simulink model "P1Ej5"  (R2022a)
settings: Solver=VariableStepAuto  StartTime=0.0  StopTime=10.0  RelTol=1e-3
settings Model: Creator=Adrian  LastModifiedBy=Adrian

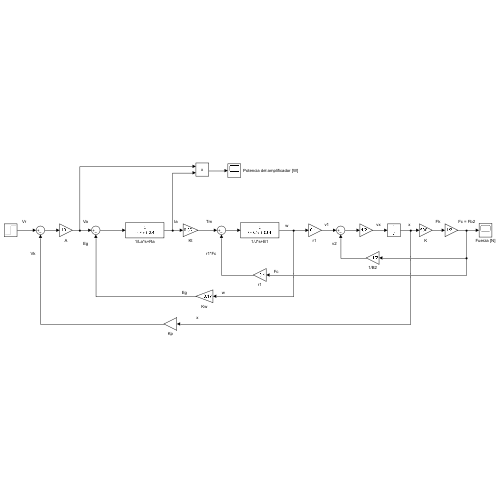
[thumbnail: Simulink's stored preview of the top-level diagram]
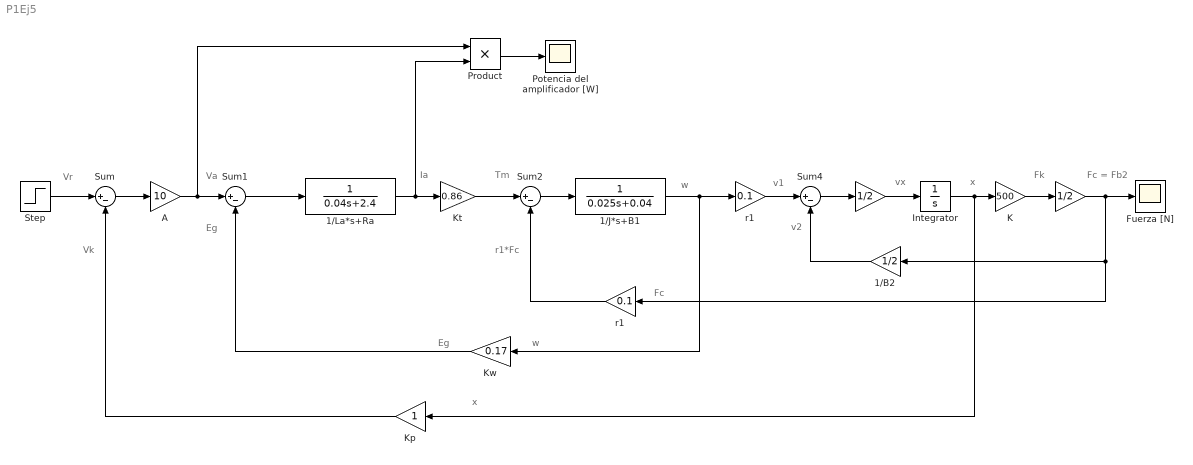
== system P1Ej5 ==
  note: vx
  note: x
  note: x
  note: v2
  note: Fk
  note: v1
  note: w
  note: Eg
  note: w
  note: Fc
  note: r1*Fc
  note: Tm
  note: Ia
  note: Eg
  note: Va
  note: Vk
  note: Fc = Fb2
  note: Vr
  " " : Gain  Gain=1/2
  "   " : Gain  Gain=1/2
  1/B2 : Gain  Gain=1/2
  1/J*s+B1 : TransferFcn  Denominator=[0.025 0.04]
  1/La*s+Ra : TransferFcn  Denominator=[0.04 2.4]
  A : Gain  Gain=10
  Fuerza [N] : Scope
  Integrator : Integrator
  K : Gain  Gain=500
  Kp : Gain
  Kt : Gain  Gain=0.86
  Kw : Gain  Gain=0.17
  Potencia del amplificador [W] : Scope
  Product : Product
  Step : Step  After=0.1725  SampleTime=0
  Sum{,1..2,4} (4 alike) : Sum  Inputs=|+-
  r1 : Gain  Gain=0.1
  "r1 " : Gain  Gain=0.1
  wires:
  Step/1 -> Sum/1
  Sum/1 -> A/1
  A/1 -> Product/1, Sum1/1
  Sum1/1 -> 1/La*s+Ra/1
  1/J*s+B1/1 -> "r1 "/1, Kw/1
  1/La*s+Ra/1 -> Product/2, Kt/1
  Kt/1 -> Sum2/1
  "   "/1 -> r1/1, 1/B2/1, Fuerza [N]/1
  Sum2/1 -> 1/J*s+B1/1
  r1/1 -> Sum2/2
  Kw/1 -> Sum1/2
  "r1 "/1 -> Sum4/1
  Sum4/1 -> " "/1
  1/B2/1 -> Sum4/2
  Kp/1 -> Sum/2
  " "/1 -> Integrator/1
  Integrator/1 -> K/1, Kp/1
  K/1 -> "   "/1
  Product/1 -> Potencia del amplificador [W]/1
